simulink model "Electon_Energization_Index_4_2"  (Simulink 10.1)
settings: Solver=ode45  StartTime=0.0  StopTime=t_stamp(end)  RelTol=1e-3  EnableMultiTasking=on
values from neighbouring files (symbols this model uses):
  Gain_factor_I1_4_2 = 1    [windmi.m]
  t_delay_E_index_4_2 = 0    [windmi.m]
undefined symbols (not defined in the file or in its folder): tau_loss_4_2
settings Model: Creator=edmund  LastModifiedBy=pavit
settings DataIOCC: TimeSaveName=tout_E  OutputSaveName=yout_E
settings DebuggingCC: UnderspecifiedInitializationDetection=Simplified  MergeDetectMultiDrivingBlocksExec=error
settings GRTTargetCC: CombineOutputUpdateFcns=on  GRTInterface=off
settings ConfigComp: CovSFcnEnable=off

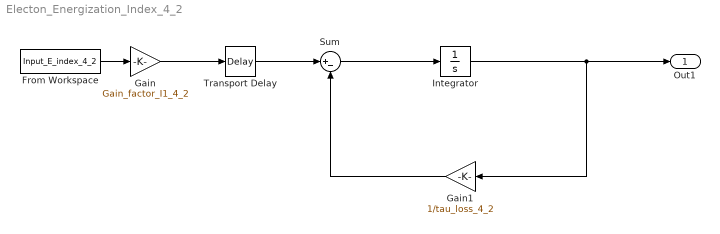
== system Electon_Energization_Index_4_2 ==
  From Workspace : FromWorkspace  VariableName=Input_E_index_4_2
  Gain : Gain  Gain=Gain_factor_I1_4_2
  Gain1 : Gain  Gain=1/tau_loss_4_2
  Integrator : Integrator
  Sum : Sum  Inputs=|+-
  Transport Delay : TransportDelay  DelayTime=t_delay_E_index_4_2
  Out1 : Outport
  wires:
  Integrator/1 -> Out1/1, Gain1/1
  Gain1/1 -> Sum/2
  From Workspace/1 -> Gain/1
  Sum/1 -> Integrator/1
  Gain/1 -> Transport Delay/1
  Transport Delay/1 -> Sum/1
